simulink model "gm_gaussianFilter"  (R2024a)
settings: Solver=FixedStepDiscrete  StartTime=0.0  StopTime=1  RelTol=1e-3
undefined symbols (not defined in the file or in its folder): G
libraries: hdlsllib x33, simulink x27, visionsources x1, visionsinks x1
(part 1 of 2)
Description:
  | Sobel Edge Detection Using the MATLAB(R) Function Block
  | This example shows how to use HDL Coder(TM) to check,
  | generate, and verify HDL code for a Sobel Edge Detection
  | block built using the MATLAB Function block.
settings Model: FPTRunName=Active  Creator=The MathWorks, Inc.  LastModifiedBy=dskap
settings SolverCC: AlgebraicLoopSolver=TrustRegion
settings DataIOCC: LimitDataPoints=on  SaveFormat=Array  SignalLogging=off  ReturnWorkspaceOutputs=off
settings OptimizationCC: BlockReduction=off  ConditionallyExecuteInputs=off  DefaultParameterBehavior=Inlined  ExpressionDepthLimit=2147483647  InitFltsAndDblsToZero=on  EfficientMapNaN2IntZero=off  LifeSpan=inf
settings DebuggingCC: AlgebraicLoopMsg=error  SaveWithParameterizedLinksMsg=none  UnderspecifiedInitializationDetection=Classic  MergeDetectMultiDrivingBlocksExec=none  SignalResolutionControl=TryResolveAllWithWarning  InheritedTsInSrcMsg=none  MultiTaskDSMMsg=warning  MultiTaskCondExecSysMsg=none  SingleTaskRateTransMsg=error  IntegerOverflowMsg=none  ParameterPrecisionLossMsg=none  FcnCallInpInsideContextMsg=warning  UnconnectedInputMsg=warning  UnconnectedOutputMsg=warning  UnconnectedLineMsg=warning  AllowSymbolicDim=off  StateNameClashWarn=warning  StrictBusMsg=ErrorOnBusTreatedAsVector  SFUnexpectedBacktrackingDiag=warning  SFNoUnconditionalDefaultTransitionDiag=warning  SFExecutionAtInitializationDiag=none  IntegerSaturationMsg=none  ArithmeticOperatorsInVariantConditions=warning
settings HardwareCC: ProdBitPerPointer=32  ProdBitPerSizeT=32  ProdBitPerPtrDiffT=32  ProdLargestAtomicFloat=None  ProdIntDivRoundTo=Undefined  ProdEndianess=Unspecified  ProdWordSize=32  ProdHWDeviceType=ASIC/FPGA  TargetHWDeviceType=32-bit Generic  ProdEqTarget=off
settings ModelReferenceCC: EnableRefExpFcnMdlSchedulingChecks=on  PropagateSignalLabelsOutOfModel=off
settings SFSimCC: SimUseLocalCustomCode=off  CustomCodeUndefinedFunction=UseInterfaceOnly
settings RTWCC: RTWUseLocalCustomCode=off  GPUComputeCapability=3.5  DLArmComputeVersion=19.05
settings CodeAppCC: StateflowObjectComments=on
settings GRTTargetCC: TargetFcnLib=ansi_tfl_tmw.mat  TargetLangStandard=C89/C90 (ANSI)  CombineOutputUpdateFcns=off  GRTInterface=on
settings ConfigComp: CovMetricSettings=dw  CovSaveCumulativeToWorkspaceVar=on  CovSaveSingleToWorkspaceVar=on  CovExternalEMLEnable=off

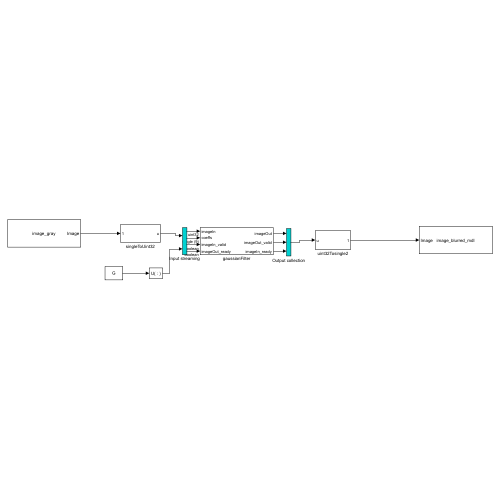
[thumbnail: Simulink's stored preview of the top-level diagram]
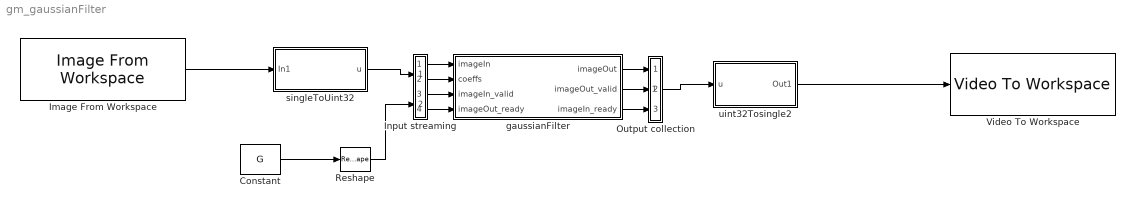
== system gm_gaussianFilter ==
  Constant : Constant  Value=G  OutDataTypeStr=single  SampleTime=-1
  Image From Workspace : visionsources/Image From Workspace  Tag=vipblks_nd  ImageValue=image_gray  Ts=1  imagePorts=One multidimensional signal  OutPortLabels=R|G|B  ImageDataType=Inherit from 'Value'  Signed=on  WordLength=16  sdImageDataType=sfix(16)  FractionLengthMode=User-defined  FractionLength=15
  Input streaming : Subsystem
      mask Display: disp('')
  Output collection : Subsystem
      mask Display: disp('')
  Reshape : Reshape
  Video To Workspace : visionsinks/Video To Workspace  VariableName=image_blurred_mdl  NumInputs=1  DataLimit=1  DecimationFactor=1  LogFi=off  InPortLabels=R|G|B
  gaussianFilter : Subsystem
  singleToUint32 : Subsystem
  uint32Tosingle2 : Subsystem
  wires:
  uint32Tosingle2/1(Out1) -> Video To Workspace/1
  Image From Workspace/1 -> singleToUint32/1(In1)
  Constant/1 -> Reshape/1
  singleToUint32/1(u) -> Input streaming/1(imageIn_orig)
  Reshape/1 -> Input streaming/2(coeffs_orig)
  Input streaming/1(imageIn) -> gaussianFilter/1(imageIn)
  Input streaming/2(coeffs) -> gaussianFilter/2(coeffs)
  Input streaming/3(imageIn_valid) -> gaussianFilter/3(imageIn_valid)
  Input streaming/4(imageOut_ready) -> gaussianFilter/4(imageOut_ready)
  Output collection/1(imageOut_orig) -> uint32Tosingle2/1(u)
  gaussianFilter/1(imageOut) -> Output collection/1(imageOut)
  gaussianFilter/2(imageOut_valid) -> Output collection/2(imageOut_valid)
  gaussianFilter/3(imageIn_ready) -> Output collection/3(imageIn_ready)

== system gm_gaussianFilter/Input streaming ==
  imageIn_orig : Inport
  coeffs_orig : Inport  Port=2
  Rate Transition : RateTransition  Integrity=off  OutPortSampleTimeOpt=Multiple of input port sample time  OutPortSampleTimeMultiple=1/360960
  coeffs_tb : MATLAB Function  TreatAsAtomicUnit=on
  imageIn_serialize : Subsystem
  imageIn_tb : MATLAB Function  TreatAsAtomicUnit=on  mask{toggleValid=off, numHighValidCycles=1, numLowValidCycles=1}
      mask prompts: toggleValid "Toggle valid signal."; numHighValidCycles "Number of valid-high signals to send between valid-low signals."; numLowValidCycles "Number of valid-low signals to send between valid-high signals."
      mask help: Control how often a 'valid' input is toggled.
  imageOut_ready_tb : MATLAB Function  TreatAsAtomicUnit=on  mask{toggleReady=off, numHighReadyCycles=1, numLowReadyCycles=1}
      mask prompts: toggleReady "Toggle ready signal."; numHighReadyCycles "Number of ready-high signals to send between ready-low signals."; numLowReadyCycles "Number of ready-low signals to send between ready-high signals."
      mask help: Control how often a 'ready' input is toggled.
  imageIn : Outport
  coeffs : Outport  Port=2
  imageIn_valid : Outport  Port=3
  imageOut_ready : Outport  Port=4
  tag scope: out_1_ready=global, valid_3=global
  wires:
  imageIn_orig/1 -> imageIn_serialize/1(In1)
  imageIn_serialize/1(Out1) -> imageIn_tb/1(imageIn_sample)
  [in_1_ready] -> imageIn_tb/2(imageIn_ready)
  imageIn_tb/1(imageIn_out_sample) -> imageIn/1
  imageIn_tb/2(imageIn_valid) -> imageIn_valid/1, [valid_3]
  coeffs_orig/1 -> Rate Transition/1
  Rate Transition/1 -> coeffs_tb/1(coeffs_in)
  [valid_3] -> coeffs_tb/2(validIn)
  coeffs_tb/1(coeffs_out) -> coeffs/1
  imageOut_ready_tb/1(imageOut_ready) -> imageOut_ready/1, [out_1_ready]

== system gm_gaussianFilter/Output collection ==
  imageOut : Inport
  imageOut_valid : Inport  Port=2
  imageIn_ready : Inport  Port=3
  AND : Logic
  imageOut_deserialize : Subsystem
  imageOut_orig : Outport
  tag scope: in_1_ready=global
  wires:
  imageOut_valid/1 -> AND/1
  [out_1_ready] -> AND/2
  imageOut/1 -> imageOut_deserialize/1(In1)
  AND/1 -> imageOut_deserialize/2(In2)
  imageOut_deserialize/1(Out1) -> imageOut_orig/1
  imageIn_ready/1 -> [in_1_ready]

== system gm_gaussianFilter/gaussianFilter ==
  imageIn : Inport  OutDataTypeStr=uint32  PortDimensions=1  SampleTime=2.77039007092199e-06
  coeffs : Inport  Port=2  OutDataTypeStr=single  PortDimensions=[9]  SampleTime=2.77039007092199e-06
  imageIn_valid : Inport  Port=3  OutDataTypeStr=boolean  SampleTime=2.77039007092199e-06
  imageOut_ready : Inport  Port=4  OutDataTypeStr=boolean  SampleTime=2.77039007092199e-06
  Input_FIFOs : Subsystem
  Output_FIFOs : Subsystem
  streaming_matrix_partition : Subsystem
  imageOut : Outport  SampleTime=2.77039007092199e-06
  imageOut_valid : Outport  Port=2  SampleTime=2.77039007092199e-06
  imageIn_ready : Outport  Port=3  SampleTime=2.77039007092199e-06
  wires:
  imageIn/1 -> Input_FIFOs/2(imageIn_in)
  coeffs/1 -> Input_FIFOs/4(coeffs_in)
  streaming_matrix_partition/1(out0) -> Output_FIFOs/2(y_in)
  imageIn_valid/1 -> Input_FIFOs/3(imageIn_valid)
  streaming_matrix_partition/2(y_valid) -> Output_FIFOs/3(y_valid_in)
  Input_FIFOs/3(imageIn_ready) -> imageIn_ready/1
  imageOut_ready/1 -> Output_FIFOs/4(y_ready)
  Input_FIFOs/5(valid) -> streaming_matrix_partition/3(in0_valid)
  Output_FIFOs/1(enable_out) -> Input_FIFOs/1(enable_in)
  Input_FIFOs/1(enable_out) -> Output_FIFOs/1(enable_in), streaming_matrix_partition/Enable
  Input_FIFOs/2(imageIn_out) -> streaming_matrix_partition/1(in0)
  Input_FIFOs/4(coeffs) -> streaming_matrix_partition/2(in1)
  Output_FIFOs/2(y_out) -> imageOut/1
  Output_FIFOs/3(y_valid) -> imageOut_valid/1

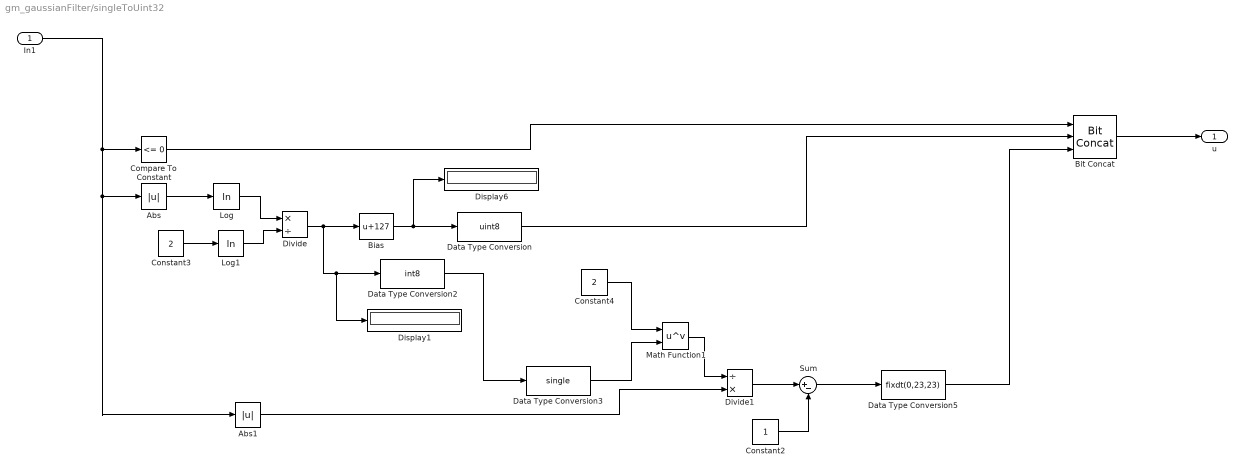
== system gm_gaussianFilter/singleToUint32 ==
  In1 : Inport
  Abs : Abs  SaturateOnIntegerOverflow=off
  Abs1 : Abs  SaturateOnIntegerOverflow=off
  Bias : Bias  Bias=127  SaturateOnIntegerOverflow=off
  Bit Concat : hdlsllib/Logic and Bit Operations/Bit Concat  numInputs=3
  Compare To Constant : simulink/Logic and Bit Operations/Compare To Constant  relop=<=  const=0  OutDataTypeStr=boolean
  Constant2 : Constant  OutDataTypeStr=single  SampleTime=-1
  Constant3 : Constant  Value=2  OutDataTypeStr=single  SampleTime=-1
  Constant4 : Constant  Value=2  OutDataTypeStr=single  SampleTime=-1
  Data Type Conversion : DataTypeConversion  OutDataTypeStr=uint8  SaturateOnIntegerOverflow=off  RndMeth=Floor
  Data Type Conversion2 : DataTypeConversion  OutDataTypeStr=int8  SaturateOnIntegerOverflow=off  RndMeth=Floor
  Data Type Conversion3 : DataTypeConversion  OutDataTypeStr=single  SaturateOnIntegerOverflow=off  RndMeth=Floor
  Data Type Conversion5 : DataTypeConversion  OutDataTypeStr=fixdt(0,23,23)  SaturateOnIntegerOverflow=off  RndMeth=Floor
  Display1 : Display
  Display6 : Display
  Divide : Product  Inputs=*/
  Divide1 : Product  Inputs=/*
  Log : Math  Operator=log
  Log1 : Math  Operator=log
  Math Function1 : Math  Operator=pow
  Sum : Sum  Inputs=|+-
  u : Outport
  wires:
  Bit Concat/1 -> u/1
  Data Type Conversion5/1 -> Bit Concat/3
  Data Type Conversion/1 -> Bit Concat/2
  Compare To Constant/1 -> Bit Concat/1
  Data Type Conversion2/1 -> Data Type Conversion3/1
  Abs1/1 -> Divide1/2
  Constant2/1 -> Sum/2
  Sum/1 -> Data Type Conversion5/1
  Divide1/1 -> Sum/1
  In1/1 -> Abs/1, Abs1/1, Compare To Constant/1
  Log/1 -> Divide/1
  Log1/1 -> Divide/2
  Math Function1/1 -> Divide1/1
  Data Type Conversion3/1 -> Math Function1/2
  Constant4/1 -> Math Function1/1
  Abs/1 -> Log/1
  Constant3/1 -> Log1/1
  Bias/1 -> Data Type Conversion/1, Display6/1
  Divide/1 -> Bias/1, Data Type Conversion2/1, Display1/1

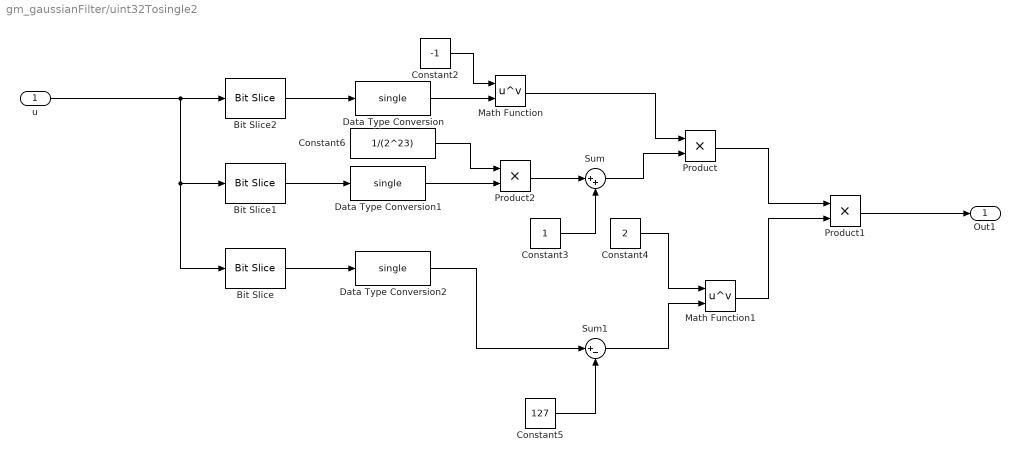
== system gm_gaussianFilter/uint32Tosingle2 ==
  u : Inport
  Bit Slice : hdlsllib/Logic and Bit Operations/Bit Slice  lidx=30  ridx=23
  Bit Slice1 : hdlsllib/Logic and Bit Operations/Bit Slice  lidx=22  ridx=0
  Bit Slice2 : hdlsllib/Logic and Bit Operations/Bit Slice  lidx=31  ridx=31
  Constant2 : Constant  Value=-1  OutDataTypeStr=single  SampleTime=-1
  Constant3 : Constant  OutDataTypeStr=single  SampleTime=-1
  Constant4 : Constant  Value=2  OutDataTypeStr=single  SampleTime=-1
  Constant5 : Constant  Value=127  OutDataTypeStr=single  SampleTime=-1
  Constant6 : Constant  Value=1/(2^23)  OutDataTypeStr=single  SampleTime=-1
  Data Type Conversion : DataTypeConversion  OutDataTypeStr=single  SaturateOnIntegerOverflow=off  RndMeth=Floor
  Data Type Conversion1 : DataTypeConversion  OutDataTypeStr=single  SaturateOnIntegerOverflow=off  RndMeth=Floor
  Data Type Conversion2 : DataTypeConversion  OutDataTypeStr=single  SaturateOnIntegerOverflow=off  RndMeth=Floor
  Math Function : Math  Operator=pow
  Math Function1 : Math  Operator=pow
  Product : Product
  Product1 : Product
  Product2 : Product
  Sum : Sum  Inputs=|++
  Sum1 : Sum  Inputs=|+-
  Out1 : Outport
  wires:
  Constant6/1 -> Product2/1
  Data Type Conversion2/1 -> Sum1/1
  Constant3/1 -> Sum/2
  Data Type Conversion1/1 -> Product2/2
  Product/1 -> Product1/1
  Sum/1 -> Product/2
  Constant2/1 -> Math Function/1
  Bit Slice/1 -> Data Type Conversion2/1
  Math Function/1 -> Product/1
  Constant5/1 -> Sum1/2
  Sum1/1 -> Math Function1/2
  Bit Slice2/1 -> Data Type Conversion/1
  Product2/1 -> Sum/1
  Constant4/1 -> Math Function1/1
  u/1 -> Bit Slice2/1, Bit Slice/1, Bit Slice1/1
  Math Function1/1 -> Product1/2
  Data Type Conversion/1 -> Math Function/2
  Bit Slice1/1 -> Data Type Conversion1/1
  Product1/1 -> Out1/1

== system gm_gaussianFilter/Input streaming/imageIn_serialize ==
  In1 : Inport
  Reshape : Reshape
  Serializer1D : hdlsllib/HDL Operations/Serializer1D  Ratio=360960  IdleCycles=0  validIn=off  startOut=off  validOut=off  inputDataDimensions=-1  inputSampleTime=-1  inputSignalType=auto
  Signal Specification : SignalSpecification  OutDataTypeStr=uint32
  Transpose : Math  Operator=transpose
  Out1 : Outport
  wires:
  In1/1 -> Transpose/1
  Transpose/1 -> Reshape/1
  Reshape/1 -> Serializer1D/1
  Serializer1D/1 -> Signal Specification/1
  Signal Specification/1 -> Out1/1

== system gm_gaussianFilter/Output collection/imageOut_deserialize ==
  In1 : Inport
  In2 : Inport  Port=2
  Deserializer1D : hdlsllib/HDL Operations/Deserializer1D  Ratio=360960  IdleCycles=0  InitialCondition=0  startIn=off  validIn=on  validOut=off  inputDataDimensions=-1  inputSampleTime=-1  inputSignalType=auto
  Reshape : Reshape  OutputDimensionality=Customize  OutputDimensions=[752 480]
  Transpose : Math  Operator=transpose
  Out1 : Outport
  wires:
  In1/1 -> Deserializer1D/1
  In2/1 -> Deserializer1D/2
  Deserializer1D/1 -> Reshape/1
  Reshape/1 -> Transpose/1
  Transpose/1 -> Out1/1

== system gm_gaussianFilter/gaussianFilter/Input_FIFOs ==
  enable_in : Inport  OutDataTypeStr=boolean  SampleTime=2.77039007092199e-06
  imageIn_in : Inport  Port=2  OutDataTypeStr=fixdt(0,32,0,'DataTypeOverride', 'Off')  SampleTime=2.77039007092199e-06
  imageIn_valid : Inport  Port=3  OutDataTypeStr=boolean  SampleTime=2.77039007092199e-06
  coeffs_in : Inport  Port=4  OutDataTypeStr=single  PortDimensions=[9 1]  SampleTime=2.77039007092199e-06
  coeffs_memory : Subsystem
  imageIn_FIFO : Subsystem
  shouldRead : Logic  AllPortsSameDT=off  OutDataTypeStr=boolean  SampleTime=2.77039007092199e-06
  enable_out : Outport  OutDataTypeStr=boolean  SampleTime=2.77039007092199e-06
  imageIn_out : Outport  Port=2  OutDataTypeStr=fixdt(0,32,0,'DataTypeOverride', 'Off')  SampleTime=2.77039007092199e-06
  imageIn_ready : Outport  Port=3  OutDataTypeStr=boolean  SampleTime=2.77039007092199e-06
  coeffs : Outport  Port=4  OutDataTypeStr=single  PortDimensions=[9 1]  SampleTime=2.77039007092199e-06
  valid : Outport  Port=5  OutDataTypeStr=boolean  SampleTime=2.77039007092199e-06
  wires:
  enable_in/1 -> shouldRead/1, enable_out/1
  shouldRead/1 -> valid/1, coeffs_memory/3(should_read), imageIn_FIFO/3(should_read)
  imageIn_in/1 -> imageIn_FIFO/1(imageIn_in)
  imageIn_valid/1 -> coeffs_memory/2(valid_in), imageIn_FIFO/2(valid_in)
  imageIn_FIFO/1(imageIn_out) -> imageIn_out/1
  imageIn_FIFO/2(imageIn_ready) -> imageIn_ready/1
  imageIn_FIFO/3(imageIn_has_data) -> shouldRead/2
  coeffs_in/1 -> coeffs_memory/1(coeffs_in)
  coeffs_memory/1(coeffs) -> coeffs/1

== system gm_gaussianFilter/gaussianFilter/Output_FIFOs ==
  enable_in : Inport  OutDataTypeStr=boolean  SampleTime=2.77039007092199e-06
  y_in : Inport  Port=2  OutDataTypeStr=fixdt(0,32,0,'DataTypeOverride', 'Off')  SampleTime=2.77039007092199e-06
  y_valid_in : Inport  Port=3  OutDataTypeStr=boolean  SampleTime=2.77039007092199e-06
  y_ready : Inport  Port=4  OutDataTypeStr=boolean  SampleTime=2.77039007092199e-06
  y_FIFO : Subsystem
  enable_out : Outport  OutDataTypeStr=boolean  SampleTime=2.77039007092199e-06
  y_out : Outport  Port=2  OutDataTypeStr=fixdt(0,32,0,'DataTypeOverride', 'Off')  SampleTime=2.77039007092199e-06
  y_valid : Outport  Port=3  OutDataTypeStr=boolean  SampleTime=2.77039007092199e-06
  wires:
  enable_in/1 -> y_FIFO/3(enable)
  y_in/1 -> y_FIFO/1(y_in)
  y_valid_in/1 -> y_FIFO/2(valid_in)
  y_ready/1 -> y_FIFO/4(ready_in)
  y_FIFO/1(y_out) -> y_out/1
  y_FIFO/2(y_valid) -> y_valid/1
  y_FIFO/3(y_has_space) -> enable_out/1

== system gm_gaussianFilter/gaussianFilter/streaming_matrix_partition ==
  in0 : Inport  OutDataTypeStr=fixdt(0,32,0,'DataTypeOverride', 'Off')  SampleTime=2.77039007092199e-06
  in1 : Inport  Port=2  OutDataTypeStr=single  PortDimensions=[9]  SampleTime=2.77039007092199e-06
  in0_valid : Inport  Port=3  OutDataTypeStr=boolean  SampleTime=2.77039007092199e-06
  enable : EnablePort  OutDataTypeStr=boolean
  Reshape : Reshape  OutputDimensionality=Customize  OutputDimensions=[3,3]
  delayMatch : Delay  DelayLength=double(197)  InitialCondition=0  SampleTime=2.77039007092199e-06
  frameBasedGaussianFilter : Subsystem
  singleToUint32 : Subsystem
  uint32Tosingle2 : Subsystem
  out0 : Outport  OutDataTypeStr=fixdt(0,32,0,'DataTypeOverride', 'Off')  SampleTime=2.77039007092199e-06
  y_valid : Outport  Port=2  OutDataTypeStr=boolean  SampleTime=2.77039007092199e-06
  wires:
  uint32Tosingle2/1(Out1) -> frameBasedGaussianFilter/1(ImageIn)
  frameBasedGaussianFilter/1(Result) -> singleToUint32/1(In1)
  Reshape/1 -> frameBasedGaussianFilter/2(data)
  singleToUint32/1(u) -> out0/1
  in0/1 -> uint32Tosingle2/1(u)
  in1/1 -> Reshape/1
  in0_valid/1 -> uint32Tosingle2/2(u_valid)
  uint32Tosingle2/2(Out1_valid) -> frameBasedGaussianFilter/3(ImageIn_valid)
  frameBasedGaussianFilter/2(Result_valid) -> singleToUint32/2(In1_valid)
  singleToUint32/2(u_valid) -> delayMatch/1
  delayMatch/1 -> y_valid/1

== system gm_gaussianFilter/gaussianFilter/Input_FIFOs/coeffs_memory ==
  coeffs_in : Inport  OutDataTypeStr=single  PortDimensions=[9 1]  SampleTime=2.77039007092199e-06
  valid_in : Inport  Port=2  OutDataTypeStr=boolean  SampleTime=2.77039007092199e-06
  should_read : Inport  Port=3  OutDataTypeStr=boolean  SampleTime=2.77039007092199e-06
  coeffs_hold : Switch  Criteria=u2 ~= 0  Threshold=double(0)  OutDataTypeStr=single  SampleTime=2.77039007092199e-06  SaturateOnIntegerOverflow=off  InputSameDT=off
  coeffs_hold_hold : Delay  DelayLength=double(1)  InitialCondition=0  SampleTime=2.77039007092199e-06
  coeffs_out : Switch  Criteria=u2 ~= 0  Threshold=double(0)  OutDataTypeStr=single  SampleTime=2.77039007092199e-06  SaturateOnIntegerOverflow=off  InputSameDT=off
  coeffs_out_hold : Delay  DelayLength=double(1)  InitialCondition=0  SampleTime=2.77039007092199e-06
  should_read_count_is_max : simulink/Logic and Bit Operations/Compare To Constant  relop===  const=double(360960)  OutDataTypeStr=boolean
  should_read_counter : hdlsllib/Sources/HDL Counter  CountType=Count limited  CountInit=double(360960)  CountStep=double(1)  CountMax=double(360960)  CountFromType=Specify  CountFrom=double(1)  CountResetPort=off  CountLoadPort=off  CountEnbPort=on  CountDirPort=off  CountHitOutputPort=off  CountDataType=Unsigned  CountWordLen=19  CountFracLen=0  CountSampTime=2.77039007092199e-06
  should_read_first : Logic  AllPortsSameDT=off  OutDataTypeStr=boolean  SampleTime=2.77039007092199e-06
  valid_in_count_is_max : simulink/Logic and Bit Operations/Compare To Constant  relop===  const=double(360960)  OutDataTypeStr=boolean
  valid_in_counter : hdlsllib/Sources/HDL Counter  CountType=Count limited  CountInit=double(360960)  CountStep=double(1)  CountMax=double(360960)  CountFromType=Specify  CountFrom=double(1)  CountResetPort=off  CountLoadPort=off  CountEnbPort=on  CountDirPort=off  CountHitOutputPort=off  CountDataType=Unsigned  CountWordLen=19  CountFracLen=0  CountSampTime=2.77039007092199e-06
  valid_in_first : Logic  AllPortsSameDT=off  OutDataTypeStr=boolean  SampleTime=2.77039007092199e-06
  coeffs : Outport  OutDataTypeStr=single  PortDimensions=[9 1]  SampleTime=2.77039007092199e-06
  wires:
  coeffs_in/1 -> coeffs_hold/1
  valid_in/1 -> valid_in_first/1, valid_in_counter/1
  should_read/1 -> should_read_first/1, should_read_counter/1
  valid_in_counter/1 -> valid_in_count_is_max/1
  valid_in_count_is_max/1 -> valid_in_first/2
  valid_in_first/1 -> coeffs_hold/2
  should_read_counter/1 -> should_read_count_is_max/1
  should_read_count_is_max/1 -> should_read_first/2
  should_read_first/1 -> coeffs_out/2
  coeffs_hold/1 -> coeffs_out/1, coeffs_hold_hold/1
  coeffs_hold_hold/1 -> coeffs_hold/3
  coeffs_out/1 -> coeffs/1, coeffs_out_hold/1
  coeffs_out_hold/1 -> coeffs_out/3

== system gm_gaussianFilter/gaussianFilter/Input_FIFOs/imageIn_FIFO ==
  imageIn_in : Inport  OutDataTypeStr=fixdt(0,32,0,'DataTypeOverride', 'Off')  SampleTime=2.77039007092199e-06
  valid_in : Inport  Port=2  OutDataTypeStr=boolean  SampleTime=2.77039007092199e-06
  should_read : Inport  Port=3  OutDataTypeStr=boolean  SampleTime=2.77039007092199e-06
  FIFO_inst : hdlsllib/HDL RAMs/HDL FIFO  fifo_size=1024  mode=FWFT  ratio=1  push_msg=Error  pop_msg=Error  show_empty=on  show_full=on  show_num=off  LabelModeActiveChoice_Mode=FWFT  rst_port=off
  hasData : Logic  Operator=NOT  Inputs=1  AllPortsSameDT=off  OutDataTypeStr=boolean  SampleTime=2.77039007092199e-06
  push : Logic  AllPortsSameDT=off  OutDataTypeStr=boolean  SampleTime=2.77039007092199e-06
  ready_out : Logic  Operator=NOT  Inputs=1  AllPortsSameDT=off  OutDataTypeStr=boolean  SampleTime=2.77039007092199e-06
  imageIn_out : Outport  OutDataTypeStr=fixdt(0,32,0,'DataTypeOverride', 'Off')  SampleTime=2.77039007092199e-06
  imageIn_ready : Outport  Port=2  OutDataTypeStr=boolean  SampleTime=2.77039007092199e-06
  imageIn_has_data : Outport  Port=3  OutDataTypeStr=boolean  SampleTime=2.77039007092199e-06
  wires:
  imageIn_in/1 -> FIFO_inst/1
  valid_in/1 -> push/1
  should_read/1 -> FIFO_inst/3
  FIFO_inst/1 -> imageIn_out/1
  FIFO_inst/2 -> hasData/1
  FIFO_inst/3 -> ready_out/1
  ready_out/1 -> imageIn_ready/1, push/2
  hasData/1 -> imageIn_has_data/1
  push/1 -> FIFO_inst/2

== system gm_gaussianFilter/gaussianFilter/Output_FIFOs/y_FIFO ==
  y_in : Inport  OutDataTypeStr=fixdt(0,32,0,'DataTypeOverride', 'Off')  SampleTime=2.77039007092199e-06
  valid_in : Inport  Port=2  OutDataTypeStr=boolean  SampleTime=2.77039007092199e-06
  enable : Inport  Port=3  OutDataTypeStr=boolean  SampleTime=2.77039007092199e-06
  ready_in : Inport  Port=4  OutDataTypeStr=boolean  SampleTime=2.77039007092199e-06
  FIFO_inst : hdlsllib/HDL RAMs/HDL FIFO  fifo_size=1024  mode=FWFT  ratio=1  push_msg=Error  pop_msg=Error  show_empty=on  show_full=on  show_num=off  LabelModeActiveChoice_Mode=FWFT  rst_port=off
  has_space : Logic  Operator=NOT  Inputs=1  AllPortsSameDT=off  OutDataTypeStr=boolean  SampleTime=2.77039007092199e-06
  pop : Logic  AllPortsSameDT=off  OutDataTypeStr=boolean  SampleTime=2.77039007092199e-06
  push : Logic  AllPortsSameDT=off  OutDataTypeStr=boolean  SampleTime=2.77039007092199e-06
  valid_out : Logic  Operator=NOT  Inputs=1  AllPortsSameDT=off  OutDataTypeStr=boolean  SampleTime=2.77039007092199e-06
  y_out : Outport  OutDataTypeStr=fixdt(0,32,0,'DataTypeOverride', 'Off')  SampleTime=2.77039007092199e-06
  y_valid : Outport  Port=2  OutDataTypeStr=boolean  SampleTime=2.77039007092199e-06
  y_has_space : Outport  Port=3  OutDataTypeStr=boolean  SampleTime=2.77039007092199e-06
  wires:
  y_in/1 -> FIFO_inst/1
  valid_in/1 -> push/1
  enable/1 -> push/2
  ready_in/1 -> pop/1
  FIFO_inst/1 -> y_out/1
  FIFO_inst/2 -> valid_out/1
  FIFO_inst/3 -> has_space/1
  valid_out/1 -> y_valid/1, pop/2
  has_space/1 -> y_has_space/1
  push/1 -> FIFO_inst/2
  pop/1 -> FIFO_inst/3

== system gm_gaussianFilter/gaussianFilter/streaming_matrix_partition/frameBasedGaussianFilter ==
  ImageIn : Inport  OutDataTypeStr=single  PortDimensions=1  SampleTime=2.77039007092199e-06
  data : Inport  Port=2  OutDataTypeStr=single  PortDimensions=[3,3]  SampleTime=2.77039007092199e-06
  ImageIn_valid : Inport  Port=3  OutDataTypeStr=boolean  SampleTime=2.77039007092199e-06
  ImageIn_NeighborhoodCreator : Subsystem
  enabledDelayMatch : Subsystem
  gaussianKernel : Subsystem
  Result : Outport  SampleTime=2.77039007092199e-06
  Result_valid : Outport  Port=2  SampleTime=2.77039007092199e-06
  wires:
  ImageIn/1 -> ImageIn_NeighborhoodCreator/1(ImageIn)
  data/1 -> enabledDelayMatch/1(data)
  gaussianKernel/1(e) -> Result/1
  ImageIn_NeighborhoodCreator/1(in_neighborhood) -> gaussianKernel/1(in)
  ImageIn_valid/1 -> enabledDelayMatch/2(ImageIn_valid), ImageIn_NeighborhoodCreator/2(ImageIn_valid)
  ImageIn_NeighborhoodCreator/2(in_neighborhood_valid) -> enabledDelayMatch/3(in_neighborhood_valid), gaussianKernel/3(in_valid)
  gaussianKernel/2(e_valid) -> Result_valid/1
  enabledDelayMatch/1(data1) -> gaussianKernel/2(data)

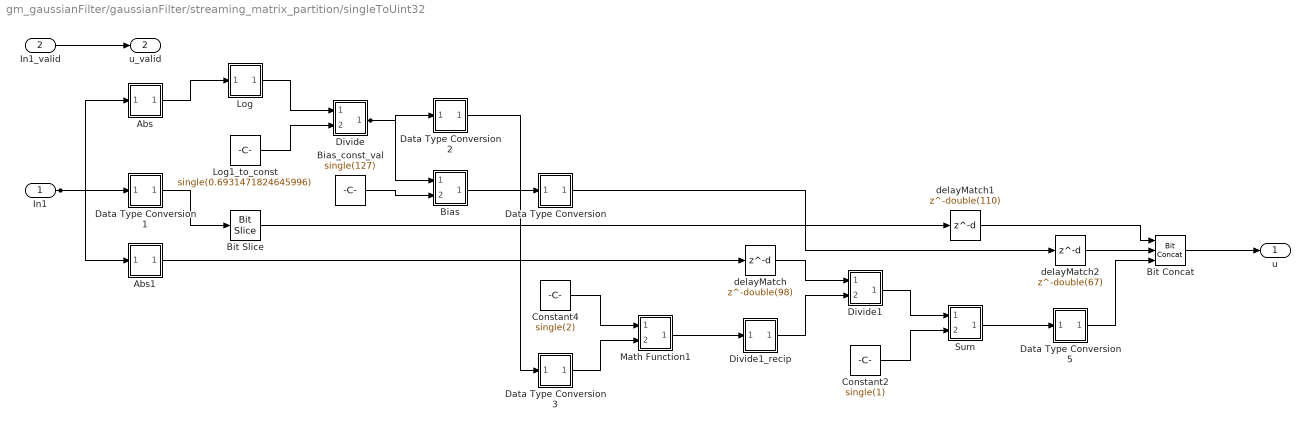
== system gm_gaussianFilter/gaussianFilter/streaming_matrix_partition/singleToUint32 ==
  In1 : Inport  OutDataTypeStr=single  PortDimensions=1  SampleTime=2.77039007092199e-06
  In1_valid : Inport  Port=2  OutDataTypeStr=boolean  SampleTime=2.77039007092199e-06
  Abs : Subsystem
      mask Display: disp('NFP\nabs');
  Abs1 : Subsystem
      mask Display: disp('NFP\nabs');
  Bias : Subsystem
      mask Display: disp('NFP\nadd');
  Bias_const_val : Constant  Value=single(127)  VectorParams1D=off  OutDataTypeStr=single  SampleTime=2.77039007092199e-06
  Bit Concat : hdlsllib/Logic and Bit Operations/Bit Concat  numInputs=3
  Bit Slice : hdlsllib/Logic and Bit Operations/Bit Slice  lidx=double(63)  ridx=double(63)
  Constant2 : Constant  Value=single(1)  OutDataTypeStr=single  SampleTime=2.77039007092199e-06
  Constant4 : Constant  Value=single(2)  OutDataTypeStr=single  SampleTime=2.77039007092199e-06
  Data Type Conversion : Subsystem
      mask Display: disp('NFP\nconv');
  Data Type Conversion1 : Subsystem
      mask Display: disp('NFP\nconv');
  Data Type Conversion2 : Subsystem
      mask Display: disp('NFP\nconv');
  Data Type Conversion3 : Subsystem
      mask Display: disp('NFP\nconv');
  Data Type Conversion5 : Subsystem
      mask Display: disp('NFP\nconv');
  Divide : Subsystem
      mask Display: disp('NFP\nmul');
  Divide1 : Subsystem
      mask Display: disp('NFP\nmul');
  Divide1_recip : Subsystem
      mask Display: disp('NFP\nmath');
  Log : Subsystem
      mask Display: disp('NFP\nmath');
  Log1_to_const : Constant  Value=single(0.6931471824645996)  OutDataTypeStr=single  SampleTime=2.77039007092199e-06
  Math Function1 : Subsystem
      mask Display: disp('NFP\nmath2');
  Sum : Subsystem
      mask Display: disp('NFP\nadd');
  delayMatch : Delay  DelayLength=double(98)  InitialCondition=0  SampleTime=2.77039007092199e-06
  delayMatch1 : Delay  DelayLength=double(110)  InitialCondition=0  SampleTime=2.77039007092199e-06
  delayMatch2 : Delay  DelayLength=double(67)  InitialCondition=0  SampleTime=2.77039007092199e-06
  u : Outport  SampleTime=2.77039007092199e-06
  u_valid : Outport  Port=2  SampleTime=2.77039007092199e-06
  wires:
  In1/1 -> Data Type Conversion1/1(In1), Abs1/1(In1), Abs/1(In1)
  Bit Concat/1 -> u/1
  delayMatch1/1 -> Bit Concat/1
  Constant2/1 -> Sum/2(In2)
  Constant4/1 -> Math Function1/1(In1)
  delayMatch2/1 -> Bit Concat/2
  Log1_to_const/1 -> Divide/2(In2)
  Bias_const_val/1 -> Bias/2(In2)
  In1_valid/1 -> u_valid/1
  Abs/1(Out1) -> Log/1(In1)
  delayMatch/1 -> Divide1/1(In1)
  Bias/1(Out1) -> Data Type Conversion/1(In1)
  Data Type Conversion/1(Out1) -> delayMatch2/1
  Data Type Conversion1/1(Out1) -> Bit Slice/1
  Data Type Conversion2/1(Out1) -> Data Type Conversion3/1(In1)
  Data Type Conversion3/1(Out1) -> Math Function1/2(In2)
  Data Type Conversion5/1(Out1) -> Bit Concat/3
  Divide/1(Out1) -> Data Type Conversion2/1(In1), Bias/1(In1)
  Divide1_recip/1(Out1) -> Divide1/2(In2)
  Divide1/1(Out1) -> Sum/1(In1)
  Log/1(Out1) -> Divide/1(In1)
  Math Function1/1(Out1) -> Divide1_recip/1(In1)
  Sum/1(Out1) -> Data Type Conversion5/1(In1)
  Abs1/1(Out1) -> delayMatch/1
  Bit Slice/1 -> delayMatch1/1

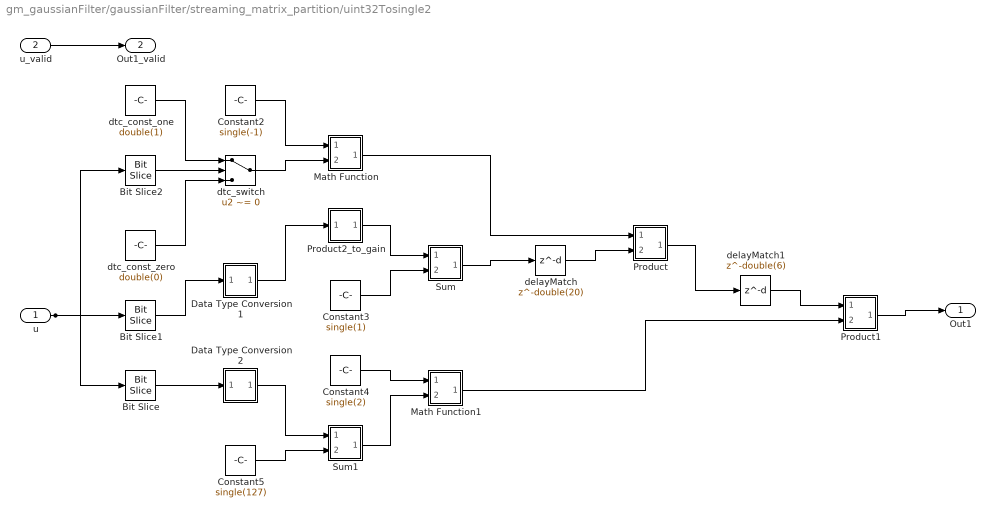
== system gm_gaussianFilter/gaussianFilter/streaming_matrix_partition/uint32Tosingle2 ==
  u : Inport  OutDataTypeStr=uint32  PortDimensions=1  SampleTime=2.77039007092199e-06
  u_valid : Inport  Port=2  OutDataTypeStr=boolean  SampleTime=2.77039007092199e-06
  Bit Slice : hdlsllib/Logic and Bit Operations/Bit Slice  lidx=double(30)  ridx=double(23)
  Bit Slice1 : hdlsllib/Logic and Bit Operations/Bit Slice  lidx=double(22)  ridx=double(0)
  Bit Slice2 : hdlsllib/Logic and Bit Operations/Bit Slice  lidx=double(31)  ridx=double(31)
  Constant2 : Constant  Value=single(-1)  OutDataTypeStr=single  SampleTime=2.77039007092199e-06
  Constant3 : Constant  Value=single(1)  OutDataTypeStr=single  SampleTime=2.77039007092199e-06
  Constant4 : Constant  Value=single(2)  OutDataTypeStr=single  SampleTime=2.77039007092199e-06
  Constant5 : Constant  Value=single(127)  OutDataTypeStr=single  SampleTime=2.77039007092199e-06
  Data Type Conversion1 : Subsystem
      mask Display: disp('NFP\nconv');
  Data Type Conversion2 : Subsystem
      mask Display: disp('NFP\nconv');
  Math Function : Subsystem
      mask Display: disp('NFP\nmath2');
  Math Function1 : Subsystem
      mask Display: disp('NFP\nmath2');
  Product : Subsystem
      mask Display: disp('NFP\nmul');
  Product1 : Subsystem
      mask Display: disp('NFP\nmul');
  Product2_to_gain : Subsystem
      mask Display: disp('NFP\ngain_pow2');
  Sum : Subsystem
      mask Display: disp('NFP\nadd');
  Sum1 : Subsystem
      mask Display: disp('NFP\nadd');
  delayMatch : Delay  DelayLength=double(20)  InitialCondition=0  SampleTime=2.77039007092199e-06
  delayMatch1 : Delay  DelayLength=double(6)  InitialCondition=0  SampleTime=2.77039007092199e-06
  dtc_const_one : Constant  Value=double(1)  OutDataTypeStr=single  SampleTime=2.77039007092199e-06
  dtc_const_zero : Constant  Value=double(0)  OutDataTypeStr=single  SampleTime=2.77039007092199e-06
  dtc_switch : Switch  Criteria=u2 ~= 0  Threshold=double(0)  OutDataTypeStr=single  SampleTime=2.77039007092199e-06  SaturateOnIntegerOverflow=off  InputSameDT=off
  Out1 : Outport  SampleTime=2.77039007092199e-06
  Out1_valid : Outport  Port=2  SampleTime=2.77039007092199e-06
  wires:
  u/1 -> Bit Slice2/1, Bit Slice1/1, Bit Slice/1
  Bit Slice/1 -> Data Type Conversion2/1(In1)
  Bit Slice1/1 -> Data Type Conversion1/1(In1)
  Bit Slice2/1 -> dtc_switch/2
  Constant2/1 -> Math Function/1(In1)
  Constant3/1 -> Sum/2(In2)
  Constant4/1 -> Math Function1/1(In1)
  Constant5/1 -> Sum1/2(In2)
  dtc_switch/1 -> Math Function/2(In2)
  delayMatch1/1 -> Product1/1(In1)
  delayMatch/1 -> Product/2(In2)
  u_valid/1 -> Out1_valid/1
  dtc_const_zero/1 -> dtc_switch/3
  dtc_const_one/1 -> dtc_switch/1
  Data Type Conversion1/1(Out1) -> Product2_to_gain/1(In1)
  Data Type Conversion2/1(Out1) -> Sum1/1(In1)
  Math Function/1(Out1) -> Product/1(In1)
  Math Function1/1(Out1) -> Product1/2(In2)
  Product/1(Out1) -> delayMatch1/1
  Product1/1(Out1) -> Out1/1
  Sum/1(Out1) -> delayMatch/1
  Sum1/1(Out1) -> Math Function1/2(In2)
  Product2_to_gain/1(Out1) -> Sum/1(In1)

== system gm_gaussianFilter/gaussianFilter/streaming_matrix_partition/frameBasedGaussianFilter/ImageIn_NeighborhoodCreator ==
  ImageIn : Inport  OutDataTypeStr=single  SampleTime=2.77039007092199e-06
  ImageIn_valid : Inport  Port=2  OutDataTypeStr=boolean  SampleTime=2.77039007092199e-06
  BoundaryCheck_3x3 : Subsystem
  NeighborhoodCreator_3x3 : Subsystem
  boundaryCounters_3_3 : Subsystem
  counterNetwork : Subsystem
  sample : Delay  DelayLength=double(1)  InitialCondition=0  SampleTime=2.77039007092199e-06
  valid : Delay  DelayLength=double(1)  InitialCondition=0  SampleTime=2.77039007092199e-06
  in_neighborhood : Outport  OutDataTypeStr=single  SampleTime=2.77039007092199e-06
  in_neighborhood_valid : Outport  Port=2  OutDataTypeStr=boolean  SampleTime=2.77039007092199e-06
  wires:
  ImageIn/1 -> sample/1
  ImageIn_valid/1 -> boundaryCounters_3_3/1(validNext), counterNetwork/1(validNext), valid/1
  sample/1 -> NeighborhoodCreator_3x3/1(sample)
  valid/1 -> boundaryCounters_3_3/2(valid), NeighborhoodCreator_3x3/2(valid), counterNetwork/2(valid)
  counterNetwork/1(isLastSample) -> boundaryCounters_3_3/3(isLastSample), NeighborhoodCreator_3x3/3(isLastSample)
  counterNetwork/2(isEndOfLine) -> boundaryCounters_3_3/4(isEndOfLine)
  counterNetwork/3(rowCtr) -> boundaryCounters_3_3/5(rowCtr)
  counterNetwork/4(colCtr) -> boundaryCounters_3_3/6(colCtr)
  counterNetwork/5(pxlCtr) -> boundaryCounters_3_3/7(pxlCtr)
  counterNetwork/6(isEndOfLineEnd) -> boundaryCounters_3_3/8(isEndOfLineEnd)
  counterNetwork/7(rowCtrEnd) -> boundaryCounters_3_3/9(rowCtrEnd)
  counterNetwork/8(colCtrEnd) -> boundaryCounters_3_3/10(colCtrEnd)
  counterNetwork/9(pxlCtrEnd) -> boundaryCounters_3_3/11(pxlCtrEnd)
  NeighborhoodCreator_3x3/1(neighborhood) -> BoundaryCheck_3x3/1(maxNeighborhood)
  boundaryCounters_3_3/1(rowCtr_3_3) -> BoundaryCheck_3x3/2(rowCtr)
  boundaryCounters_3_3/2(colCtr_3_3) -> BoundaryCheck_3x3/3(colCtr)
  boundaryCounters_3_3/3(shift_3_3) -> BoundaryCheck_3x3/4(shift)
  boundaryCounters_3_3/4(valid_3_3) -> in_neighborhood_valid/1
  BoundaryCheck_3x3/1(neighborhood_3x3) -> in_neighborhood/1

== system gm_gaussianFilter/gaussianFilter/streaming_matrix_partition/frameBasedGaussianFilter/enabledDelayMatch ==
  data : Inport  OutDataTypeStr=single  SampleTime=2.77039007092199e-06
  ImageIn_valid : Inport  Port=2  OutDataTypeStr=boolean  SampleTime=2.77039007092199e-06
  in_neighborhood_valid : Inport  Port=3  OutDataTypeStr=boolean  SampleTime=2.77039007092199e-06
  data_hold : Switch  Criteria=u2 ~= 0  Threshold=double(0)  OutDataTypeStr=single  SampleTime=2.77039007092199e-06  SaturateOnIntegerOverflow=off  InputSameDT=off
  data_next : Delay  DelayLength=double(1)  InitialCondition=0  SampleTime=2.77039007092199e-06
  data_out : Switch  Criteria=u2 ~= 0  Threshold=double(0)  OutDataTypeStr=single  SampleTime=2.77039007092199e-06  SaturateOnIntegerOverflow=off  InputSameDT=off
  data_out_hold : Delay  DelayLength=double(1)  InitialCondition=0  SampleTime=2.77039007092199e-06
  delayMatch : Delay  DelayLength=double(1)  InitialCondition=0  SampleTime=2.77039007092199e-06
  enbFinalDelay : Logic  AllPortsSameDT=off  OutDataTypeStr=boolean  SampleTime=2.77039007092199e-06
  enbInitialDelay : Logic  AllPortsSameDT=off  OutDataTypeStr=boolean  SampleTime=2.77039007092199e-06
  firstReadSample : simulink/Logic and Bit Operations/Compare To Constant  relop===  const=double(1)  OutDataTypeStr=boolean
  firstWrittenSample : simulink/Logic and Bit Operations/Compare To Constant  relop===  const=double(1)  OutDataTypeStr=boolean
  frameReadCtr : hdlsllib/Sources/HDL Counter  CountType=Count limited  CountInit=double(1)  CountStep=double(1)  CountMax=double(360960)  CountFromType=Initial value  CountFrom=double(1)  CountResetPort=off  CountLoadPort=off  CountEnbPort=on  CountDirPort=off  CountHitOutputPort=off  CountDataType=Unsigned  CountWordLen=19  CountFracLen=0  CountSampTime=2.77039007092199e-06
  frameWriteCtr : hdlsllib/Sources/HDL Counter  CountType=Count limited  CountInit=double(1)  CountStep=double(1)  CountMax=double(360960)  CountFromType=Initial value  CountFrom=double(1)  CountResetPort=off  CountLoadPort=off  CountEnbPort=on  CountDirPort=off  CountHitOutputPort=off  CountDataType=Unsigned  CountWordLen=19  CountFracLen=0  CountSampTime=2.77039007092199e-06
  t : Reshape  OutputDimensionality=Column vector (2-D)
  t1 : Reshape  OutputDimensionality=Column vector (2-D)
  t2 : Reshape  OutputDimensionality=Customize  OutputDimensions=[3,3]
  data1 : Outport  OutDataTypeStr=single  SampleTime=2.77039007092199e-06
  wires:
  data/1 -> t/1
  ImageIn_valid/1 -> enbInitialDelay/2, frameWriteCtr/1
  in_neighborhood_valid/1 -> enbFinalDelay/2, frameReadCtr/1
  frameWriteCtr/1 -> firstWrittenSample/1
  firstWrittenSample/1 -> enbInitialDelay/1
  enbInitialDelay/1 -> data_hold/2
  frameReadCtr/1 -> firstReadSample/1
  firstReadSample/1 -> enbFinalDelay/1
  enbFinalDelay/1 -> data_out/2
  t/1 -> data_hold/1
  delayMatch/1 -> data_out/1
  data_next/1 -> delayMatch/1, data_hold/3
  data_hold/1 -> data_next/1
  t2/1 -> t1/1, data1/1
  t1/1 -> data_out_hold/1
  data_out_hold/1 -> data_out/3
  data_out/1 -> t2/1

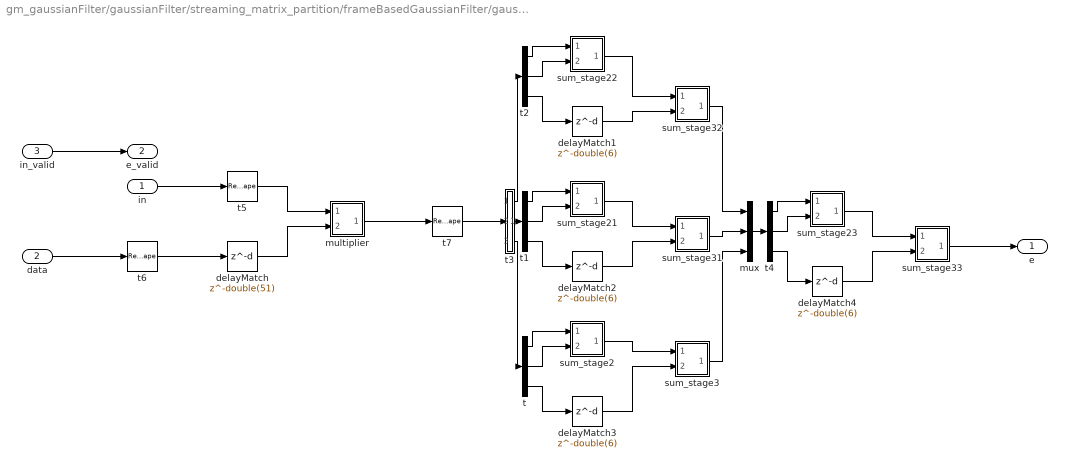
== system gm_gaussianFilter/gaussianFilter/streaming_matrix_partition/frameBasedGaussianFilter/gaussianKernel ==
  in : Inport  OutDataTypeStr=single  SampleTime=2.77039007092199e-06
  data : Inport  Port=2  OutDataTypeStr=single  SampleTime=2.77039007092199e-06
  in_valid : Inport  Port=3  OutDataTypeStr=boolean  SampleTime=2.77039007092199e-06
  delayMatch : Delay  DelayLength=double(51)  InitialCondition=0  SampleTime=2.77039007092199e-06
  delayMatch{1..4} (4 alike) : Delay  DelayLength=double(6)  InitialCondition=0  SampleTime=2.77039007092199e-06
  multiplier : Subsystem
      mask Display: disp('NFP\nmul');
  mux : Mux  Inputs=3
  sum_stage2 : Subsystem
      mask Display: disp('NFP\nadd');
  sum_stage21 : Subsystem
      mask Display: disp('NFP\nadd');
  sum_stage22 : Subsystem
      mask Display: disp('NFP\nadd');
  sum_stage23 : Subsystem
      mask Display: disp('NFP\nadd');
  sum_stage3 : Subsystem
      mask Display: disp('NFP\nadd');
  sum_stage31 : Subsystem
      mask Display: disp('NFP\nadd');
  sum_stage32 : Subsystem
      mask Display: disp('NFP\nadd');
  sum_stage33 : Subsystem
      mask Display: disp('NFP\nadd');
  t{,1..2,4} (4 alike) : Demux  Outputs=3
  t3 : Subsystem
  t5 : Reshape  OutputDimensionality=Column vector (2-D)
  t6 : Reshape  OutputDimensionality=Column vector (2-D)
  t7 : Reshape  OutputDimensionality=Customize  OutputDimensions=[3,3]
  e : Outport  OutDataTypeStr=single  SampleTime=2.77039007092199e-06
  e_valid : Outport  Port=2  OutDataTypeStr=boolean  SampleTime=2.77039007092199e-06
  wires:
  in/1 -> t5/1
  data/1 -> t6/1
  t7/1 -> t3/1(in0)
  mux/1 -> t4/1
  delayMatch3/1 -> sum_stage3/2(In2)
  delayMatch2/1 -> sum_stage31/2(In2)
  delayMatch1/1 -> sum_stage32/2(In2)
  t3/3(out2) -> t/1
  t/2 -> sum_stage2/2(In2)
  t/1 -> sum_stage2/1(In1)
  t3/2(out1) -> t1/1
  t1/2 -> sum_stage21/2(In2)
  t1/1 -> sum_stage21/1(In1)
  t3/1(out0) -> t2/1
  t2/2 -> sum_stage22/2(In2)
  t2/1 -> sum_stage22/1(In1)
  delayMatch4/1 -> sum_stage33/2(In2)
  t4/2 -> sum_stage23/2(In2)
  t4/1 -> sum_stage23/1(In1)
  in_valid/1 -> e_valid/1
  t5/1 -> multiplier/1(In1)
  delayMatch/1 -> multiplier/2(In2)
  multiplier/1(Out1) -> t7/1
  sum_stage3/1(Out1) -> mux/3
  sum_stage31/1(Out1) -> mux/2
  sum_stage32/1(Out1) -> mux/1
  sum_stage2/1(Out1) -> sum_stage3/1(In1)
  sum_stage21/1(Out1) -> sum_stage31/1(In1)
  sum_stage22/1(Out1) -> sum_stage32/1(In1)
  sum_stage33/1(Out1) -> e/1
  sum_stage23/1(Out1) -> sum_stage33/1(In1)
  t6/1 -> delayMatch/1
  t2/3 -> delayMatch1/1
  t1/3 -> delayMatch2/1
  t/3 -> delayMatch3/1
  t4/3 -> delayMatch4/1

== system gm_gaussianFilter/gaussianFilter/streaming_matrix_partition/singleToUint32/Abs ==
  In1 : Inport
  Abs : Abs  SampleTime=2.77039007092199e-06  OutDataTypeStr=single  SaturateOnIntegerOverflow=off
  Out1 : Outport
  wires:
  In1/1 -> Abs/1
  Abs/1 -> Out1/1

== system gm_gaussianFilter/gaussianFilter/streaming_matrix_partition/singleToUint32/Abs1 ==
  In1 : Inport
  Abs1 : Abs  SampleTime=2.77039007092199e-06  OutDataTypeStr=single  SaturateOnIntegerOverflow=off
  Out1 : Outport
  wires:
  In1/1 -> Abs1/1
  Abs1/1 -> Out1/1

== system gm_gaussianFilter/gaussianFilter/streaming_matrix_partition/singleToUint32/Bias ==
  In1 : Inport
  In2 : Inport  Port=2
  Bias : Sum  OutDataTypeStr=single  RndMeth=Nearest  SampleTime=2.77039007092199e-06
  Bias_pd1 : Delay  DelayLength=6
  Out1 : Outport
  wires:
  In1/1 -> Bias/1
  In2/1 -> Bias/2
  Bias/1 -> Bias_pd1/1
  Bias_pd1/1 -> Out1/1

== system gm_gaussianFilter/gaussianFilter/streaming_matrix_partition/singleToUint32/Data Type Conversion ==
  In1 : Inport
  Data Type Conversion : DataTypeConversion  OutDataTypeStr=uint8  SampleTime=2.77039007092199e-06  SaturateOnIntegerOverflow=off  RndMeth=Floor
  Data Type Conversion_pd1 : Delay  DelayLength=6
  Out1 : Outport
  wires:
  In1/1 -> Data Type Conversion/1
  Data Type Conversion/1 -> Data Type Conversion_pd1/1
  Data Type Conversion_pd1/1 -> Out1/1

== system gm_gaussianFilter/gaussianFilter/streaming_matrix_partition/singleToUint32/Data Type Conversion1 ==
  In1 : Inport
  Data Type Conversion1 : DataTypeConversion  OutDataTypeStr=fixdt(1, 64, 0)  SampleTime=2.77039007092199e-06  SaturateOnIntegerOverflow=off  RndMeth=Floor
  Data Type Conversion1_pd1 : Delay  DelayLength=6
  Out1 : Outport
  wires:
  In1/1 -> Data Type Conversion1/1
  Data Type Conversion1/1 -> Data Type Conversion1_pd1/1
  Data Type Conversion1_pd1/1 -> Out1/1

== system gm_gaussianFilter/gaussianFilter/streaming_matrix_partition/singleToUint32/Data Type Conversion2 ==
  In1 : Inport
  Data Type Conversion2 : DataTypeConversion  OutDataTypeStr=int8  SampleTime=2.77039007092199e-06  SaturateOnIntegerOverflow=off  RndMeth=Floor
  Data Type Conversion2_pd1 : Delay  DelayLength=6
  Out1 : Outport
  wires:
  In1/1 -> Data Type Conversion2/1
  Data Type Conversion2/1 -> Data Type Conversion2_pd1/1
  Data Type Conversion2_pd1/1 -> Out1/1

== system gm_gaussianFilter/gaussianFilter/streaming_matrix_partition/singleToUint32/Data Type Conversion3 ==
  In1 : Inport
  Data Type Conversion3 : DataTypeConversion  OutDataTypeStr=single  SampleTime=2.77039007092199e-06  SaturateOnIntegerOverflow=off  RndMeth=Floor
  Data Type Conversion3_pd1 : Delay  DelayLength=6
  Out1 : Outport
  wires:
  In1/1 -> Data Type Conversion3/1
  Data Type Conversion3/1 -> Data Type Conversion3_pd1/1
  Data Type Conversion3_pd1/1 -> Out1/1

== system gm_gaussianFilter/gaussianFilter/streaming_matrix_partition/singleToUint32/Data Type Conversion5 ==
  In1 : Inport
  Data Type Conversion5 : DataTypeConversion  OutDataTypeStr=fixdt(0, 23, 23)  SampleTime=2.77039007092199e-06  SaturateOnIntegerOverflow=off  RndMeth=Floor
  Data Type Conversion5_pd1 : Delay  DelayLength=6
  Out1 : Outport
  wires:
  In1/1 -> Data Type Conversion5/1
  Data Type Conversion5/1 -> Data Type Conversion5_pd1/1
  Data Type Conversion5_pd1/1 -> Out1/1

== system gm_gaussianFilter/gaussianFilter/streaming_matrix_partition/singleToUint32/Divide ==
  In1 : Inport
  In2 : Inport  Port=2
  Divide : Product  Inputs=*/  OutDataTypeStr=single  SampleTime=2.77039007092199e-06
  Divide_pd1 : Delay  DelayLength=17
  Out1 : Outport
  wires:
  In1/1 -> Divide/1
  In2/1 -> Divide/2
  Divide/1 -> Divide_pd1/1
  Divide_pd1/1 -> Out1/1

== system gm_gaussianFilter/gaussianFilter/streaming_matrix_partition/singleToUint32/Divide1 ==
  In1 : Inport
  In2 : Inport  Port=2
  Divide1 : Product  Inputs=**  OutDataTypeStr=single  SampleTime=2.77039007092199e-06
  Divide1_pd1 : Delay  DelayLength=6
  Out1 : Outport
  wires:
  In1/1 -> Divide1/1
  In2/1 -> Divide1/2
  Divide1/1 -> Divide1_pd1/1
  Divide1_pd1/1 -> Out1/1

== system gm_gaussianFilter/gaussianFilter/streaming_matrix_partition/singleToUint32/Divide1_recip ==
  In1 : Inport
  Divide1_recip : Math  Operator=reciprocal  SampleTime=2.77039007092199e-06
  Divide1_recip_pd1 : Delay  DelayLength=16
  Out1 : Outport
  wires:
  In1/1 -> Divide1_recip/1
  Divide1_recip/1 -> Divide1_recip_pd1/1
  Divide1_recip_pd1/1 -> Out1/1

== system gm_gaussianFilter/gaussianFilter/streaming_matrix_partition/singleToUint32/Log ==
  In1 : Inport
  Log : Math  Operator=log  SampleTime=2.77039007092199e-06
  Log_pd1 : Delay  DelayLength=20
  Out1 : Outport
  wires:
  In1/1 -> Log/1
  Log/1 -> Log_pd1/1
  Log_pd1/1 -> Out1/1

== system gm_gaussianFilter/gaussianFilter/streaming_matrix_partition/singleToUint32/Math Function1 ==
  In1 : Inport
  In2 : Inport  Port=2
  Math Function1 : Math  Operator=pow  SampleTime=2.77039007092199e-06
  Math Function1_pd1 : Delay  DelayLength=33
  Out1 : Outport
  wires:
  In1/1 -> Math Function1/1
  In2/1 -> Math Function1/2
  Math Function1/1 -> Math Function1_pd1/1
  Math Function1_pd1/1 -> Out1/1

== system gm_gaussianFilter/gaussianFilter/streaming_matrix_partition/singleToUint32/Sum ==
  In1 : Inport
  In2 : Inport  Port=2
  Sum : Sum  Inputs=+-  OutDataTypeStr=single  SampleTime=2.77039007092199e-06
  Sum_pd1 : Delay  DelayLength=6
  Out1 : Outport
  wires:
  In1/1 -> Sum/1
  In2/1 -> Sum/2
  Sum/1 -> Sum_pd1/1
  Sum_pd1/1 -> Out1/1

== system gm_gaussianFilter/gaussianFilter/streaming_matrix_partition/uint32Tosingle2/Data Type Conversion1 ==
  In1 : Inport
  Data Type Conversion1 : DataTypeConversion  OutDataTypeStr=single  SampleTime=2.77039007092199e-06  SaturateOnIntegerOverflow=off  RndMeth=Floor
  Data Type Conversion1_pd1 : Delay  DelayLength=6
  Out1 : Outport
  wires:
  In1/1 -> Data Type Conversion1/1
  Data Type Conversion1/1 -> Data Type Conversion1_pd1/1
  Data Type Conversion1_pd1/1 -> Out1/1

== system gm_gaussianFilter/gaussianFilter/streaming_matrix_partition/uint32Tosingle2/Data Type Conversion2 ==
  In1 : Inport
  Data Type Conversion2 : DataTypeConversion  OutDataTypeStr=single  SampleTime=2.77039007092199e-06  SaturateOnIntegerOverflow=off  RndMeth=Floor
  Data Type Conversion2_pd1 : Delay  DelayLength=6
  Out1 : Outport
  wires:
  In1/1 -> Data Type Conversion2/1
  Data Type Conversion2/1 -> Data Type Conversion2_pd1/1
  Data Type Conversion2_pd1/1 -> Out1/1

== system gm_gaussianFilter/gaussianFilter/streaming_matrix_partition/uint32Tosingle2/Math Function ==
  In1 : Inport
  In2 : Inport  Port=2
  Math Function : Math  Operator=pow  SampleTime=2.77039007092199e-06
  Math Function_pd1 : Delay  DelayLength=33
  Out1 : Outport
  wires:
  In1/1 -> Math Function/1
  In2/1 -> Math Function/2
  Math Function/1 -> Math Function_pd1/1
  Math Function_pd1/1 -> Out1/1

== system gm_gaussianFilter/gaussianFilter/streaming_matrix_partition/uint32Tosingle2/Math Function1 ==
  In1 : Inport
  In2 : Inport  Port=2
  Math Function1 : Math  Operator=pow  SampleTime=2.77039007092199e-06
  Math Function1_pd1 : Delay  DelayLength=33
  Out1 : Outport
  wires:
  In1/1 -> Math Function1/1
  In2/1 -> Math Function1/2
  Math Function1/1 -> Math Function1_pd1/1
  Math Function1_pd1/1 -> Out1/1

== system gm_gaussianFilter/gaussianFilter/streaming_matrix_partition/uint32Tosingle2/Product ==
  In1 : Inport
  In2 : Inport  Port=2
  Product : Product  Inputs=**  OutDataTypeStr=single  SampleTime=2.77039007092199e-06
  Product_pd1 : Delay  DelayLength=6
  Out1 : Outport
  wires:
  In1/1 -> Product/1
  In2/1 -> Product/2
  Product/1 -> Product_pd1/1
  Product_pd1/1 -> Out1/1

== system gm_gaussianFilter/gaussianFilter/streaming_matrix_partition/uint32Tosingle2/Product1 ==
  In1 : Inport
  In2 : Inport  Port=2
  Product1 : Product  Inputs=**  OutDataTypeStr=single  SampleTime=2.77039007092199e-06
  Product1_pd1 : Delay  DelayLength=6
  Out1 : Outport
  wires:
  In1/1 -> Product1/1
  In2/1 -> Product1/2
  Product1/1 -> Product1_pd1/1
  Product1_pd1/1 -> Out1/1

== system gm_gaussianFilter/gaussianFilter/streaming_matrix_partition/uint32Tosingle2/Product2_to_gain ==
  In1 : Inport
  Product2_to_gain : Gain  Gain=single(1.1920928955078125e-07)
  Product2_to_gain_pd1 : Delay  DelayLength=1
  Out1 : Outport
  wires:
  In1/1 -> Product2_to_gain/1
  Product2_to_gain/1 -> Product2_to_gain_pd1/1
  Product2_to_gain_pd1/1 -> Out1/1

== system gm_gaussianFilter/gaussianFilter/streaming_matrix_partition/uint32Tosingle2/Sum ==
  In1 : Inport
  In2 : Inport  Port=2
  Sum : Sum  OutDataTypeStr=single  SampleTime=2.77039007092199e-06
  Sum_pd1 : Delay  DelayLength=6
  Out1 : Outport
  wires:
  In1/1 -> Sum/1
  In2/1 -> Sum/2
  Sum/1 -> Sum_pd1/1
  Sum_pd1/1 -> Out1/1

== system gm_gaussianFilter/gaussianFilter/streaming_matrix_partition/uint32Tosingle2/Sum1 ==
  In1 : Inport
  In2 : Inport  Port=2
  Sum1 : Sum  Inputs=+-  OutDataTypeStr=single  SampleTime=2.77039007092199e-06
  Sum1_pd1 : Delay  DelayLength=6
  Out1 : Outport
  wires:
  In1/1 -> Sum1/1
  In2/1 -> Sum1/2
  Sum1/1 -> Sum1_pd1/1
  Sum1_pd1/1 -> Out1/1
